simulink library "MainLibrary"  (R2023a)
settings: Solver=VariableStepAuto  StartTime=0.0  StopTime=10.0  RelTol=1e-3
undefined symbols (not defined in the file or in its folder): baseRate
libraries: simulink x1
settings Model: Creator=AlexC  LastModifiedBy=SPOT
settings SolverCC: AlgebraicLoopSolver=TrustRegion
settings DataIOCC: ReturnWorkspaceOutputs=off
settings DebuggingCC: UnconnectedInputMsg=warning  UnconnectedOutputMsg=warning  UnconnectedLineMsg=warning  ArithmeticOperatorsInVariantConditions=warning
settings ModelReferenceCC: EnableRefExpFcnMdlSchedulingChecks=on
settings SFSimCC: SimUseLocalCustomCode=off  CustomCodeUndefinedFunction=UseInterfaceOnly
settings RTWCC: RTWUseLocalCustomCode=off

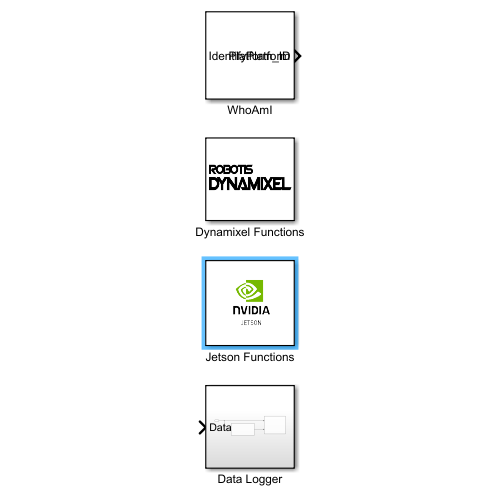
[thumbnail: Simulink's stored preview of the top-level diagram]
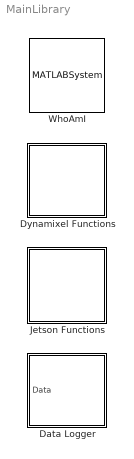
== system MainLibrary ==
  Data Logger : Subsystem
  Dynamixel Functions : Subsystem
      mask Display: image('$imagefile'); % Use "Edit Image" on toolstrip to change.
  Jetson Functions : Subsystem
      mask Display: image('$imagefile'); % Use "Edit Image" on toolstrip to change.
  WhoAmI : MATLABSystem  System=IdentifyPlatform  SampleTime=0.1
      mask Type: IdentifyPlatform
      mask Display:
      | disp('IdentifyPlatform');
      | port_label('output',1,'Platform_ID');

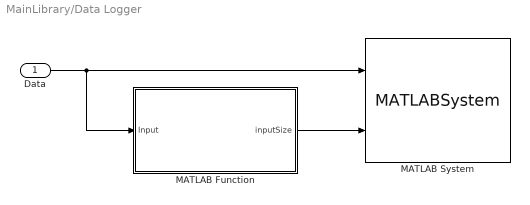
== system MainLibrary/Data Logger ==
  Data : Inport
  MATLAB Function : MATLAB Function  TreatAsAtomicUnit=on
  MATLAB System : MATLABSystem  System=CustomDataLogger
      mask Type: CustomDataLogger
      mask Display:
      | disp('CustomDataLogger');
      | port_label('input',1,'u1');
      | port_label('input',2,'u2');
  wires:
  Data/1 -> MATLAB Function/1(Input), MATLAB System/1
  MATLAB Function/1(inputSize) -> MATLAB System/2

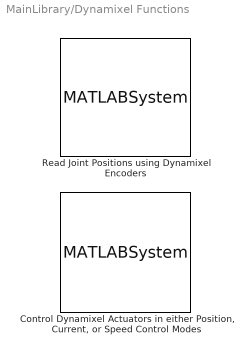
== system MainLibrary/Dynamixel Functions ==
  "Control Dynamixel Actuators in either Position, Current, or Speed Control Modes" : MATLABSystem  System=Dynamixel_Controller  POSITION_P_GAIN=400  POSITION_I_GAIN=0  POSITION_D_GAIN=200  MAX_POSITION=3072  MIN_POSITION=1024  MOVE_TIME=0  CURRENT_LIMIT=850  SPEED_P_GAIN=100  SPEED_I_GAIN=1920  VELOCITY_LIMIT=1023  ACCELERATION_TIME=0  SampleTime=baseRate
      mask Type: Dynamixel_Controller
      mask Display:
      | disp('Dynamixel_Controller');
      | port_label('input',1,'Control_Mode');
      | port_label('input',2,'Joint1_Command');
      | port_label('input',3,'Joint2_Command');
      | port_label('input',4,'Joint3_Command');
  Read Joint Positions using Dynamixel Encoders : MATLABSystem  System=ReadArm_Position_Rates  SampleTime=baseRate
      mask Type: ReadArm_Position_Rates
      mask Display:
      | disp('ReadArm_Position_Rates');
      | port_label('input',1,'u1');
      | port_label('input',2,'u2');
      | port_label('input',3,'u3');
      | port_label('output',1,'theta1');
      | port_label('output',2,'theta2');
      | port_label('output',3,'theta3');
      | port_label('output',4,'omega1');
      | port_label('output',5,'omega2');
      | port_label('output',6,'omega3');

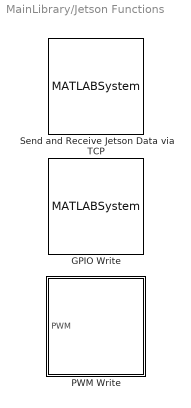
== system MainLibrary/Jetson Functions ==
  GPIO Write : MATLABSystem  System=GPIO_Write  gpioPin=428  pinDirection=1
      mask Type: GPIO_Write
      mask Display:
      | disp('GPIO_Write');
      | port_label('input',1,'u');
  PWM Write : Subsystem  mask{Set_GPIO=0}
      mask prompts: Set_GPIO "GPIO Pin"
      mask DialogControl DescGroupVar Prompt: PWM Control
      mask DialogControl DescTextVar Prompt: Select which GPIO you would like to control via software PWM.
  Send and Receive Jetson Data via TCP : MATLABSystem  System=guidance_server
      mask Type: guidance_server
      mask Display: disp('guidance_server');

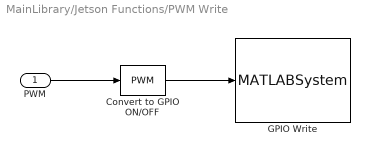
== system MainLibrary/Jetson Functions/PWM Write ==
  PWM : Inport
  Convert to GPIO ON/OFF : simulink/Discontinuities/PWM  DisableCoverage=on  Period=0.1  InitialDelay=0  DisallowZeroDutyCycle=off  RunAtFixedTimeIntervals=on  SampleTime=baseRate
  GPIO Write : MATLABSystem  System=GPIO_Write  gpioPin=480  pinDirection=1
      mask Type: GPIO_Write
      mask Display:
      | disp('GPIO_Write');
      | port_label('input',1,'u');
  wires:
  Convert to GPIO ON/OFF/1 -> GPIO Write/1
  PWM/1 -> Convert to GPIO ON/OFF/1

== matlab function MainLibrary/Data Logger/MATLAB Function ==
  data: Input input; inputSize output
function inputSize = getSizeInput(Input)

    inputSize = max(size(Input));

end
